simulink library "INT_CEngDsT_VDDynTst"  (R2016b)
settings: Solver=VariableStepAuto  StartTime=0.0  StopTime=10.0  RelTol=1e-3
settings Model: Creator=lenovo  LastModifiedBy=lenovo

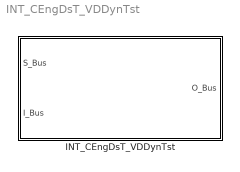
== system INT_CEngDsT_VDDynTst ==
  INT_CEngDsT_VDDynTst : Subsystem

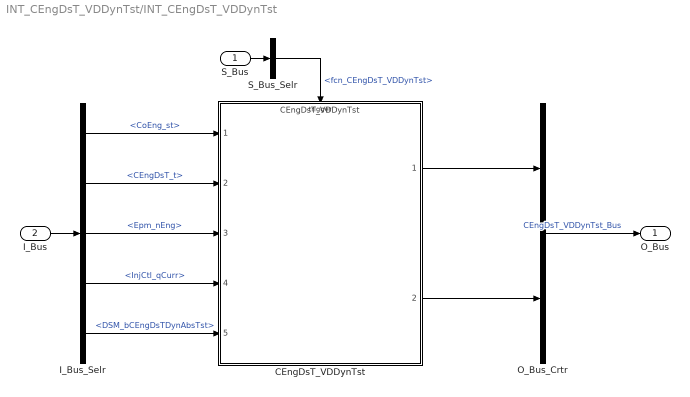
== system INT_CEngDsT_VDDynTst/INT_CEngDsT_VDDynTst ==
  S_Bus : Inport
  I_Bus : Inport  Port=2
  CEngDsT_VDDynTst : ModelReference  ModelNameDialog=CEngDsT_VDDynTst  ModelReferenceVersion=1.5  TriggerPortName=function  TriggerPortTriggerType=function-call  TriggerPortStatesWhenEnabling=held
  I_Bus_Selr : BusSelector  OutputSignals=CoEng_st,CEngDsT_t,Epm_nEng,InjCtl_qCurr,DSM_bCEngDsTDynAbsTst
  O_Bus_Crtr : BusCreator  Inputs=2
  S_Bus_Selr : BusSelector  OutputSignals=fcn_CEngDsT_VDDynTst
  O_Bus : Outport
  wires:
  S_Bus_Selr/1 -> CEngDsT_VDDynTst/Trigger  "<fcn_CEngDsT_VDDynTst>"
  S_Bus/1 -> S_Bus_Selr/1
  I_Bus/1 -> I_Bus_Selr/1
  I_Bus_Selr/1 -> CEngDsT_VDDynTst/1  "<CoEng_st>"
  I_Bus_Selr/2 -> CEngDsT_VDDynTst/2  "<CEngDsT_t>"
  I_Bus_Selr/3 -> CEngDsT_VDDynTst/3  "<Epm_nEng>"
  I_Bus_Selr/4 -> CEngDsT_VDDynTst/4  "<InjCtl_qCurr>"
  I_Bus_Selr/5 -> CEngDsT_VDDynTst/5  "<DSM_bCEngDsTDynAbsTst>"
  O_Bus_Crtr/1 -> O_Bus/1  "CEngDsT_VDDynTst_Bus"
  CEngDsT_VDDynTst/1 -> O_Bus_Crtr/1
  CEngDsT_VDDynTst/2 -> O_Bus_Crtr/2
